simulink model "exampleThermalConductivity"  (Simulink 7.6)
settings: Solver=ode45  StartTime=0.0  StopTime=10.0  RelTol=1e-3
libraries: carnot x4
settings Model: Creator=drhf  LastModifiedBy=drhf

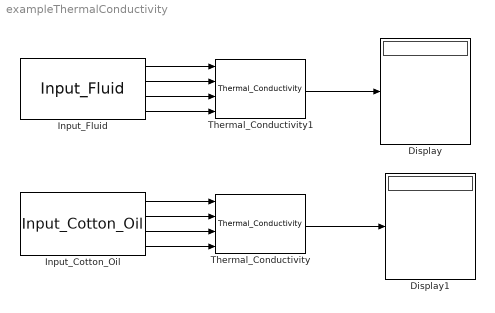
== system exampleThermalConductivity ==
  Display : Display
  Display1 : Display
  Input_Cotton_Oil : carnot/Basic/Material_Properties/Input_Cotton_Oil  SystemSampleTime=-1  T=[10:10:50]  p=1e5
  Input_Fluid : carnot/Basic/Material_Properties/Input_Fluid  SystemSampleTime=-1  fluid=water  T=[10:10:50]  p=1e5  x=0.005
  Thermal_Conductivity : carnot/Basic/Material_Properties/Thermal_Conductivity  SystemSampleTime=-1
  Thermal_Conductivity1 : carnot/Basic/Material_Properties/Thermal_Conductivity  SystemSampleTime=-1
  wires:
  Input_Fluid/1 -> Thermal_Conductivity1/1
  Input_Fluid/2 -> Thermal_Conductivity1/2
  Input_Fluid/3 -> Thermal_Conductivity1/3
  Input_Fluid/4 -> Thermal_Conductivity1/4
  Thermal_Conductivity1/1 -> Display/1
  Input_Cotton_Oil/1 -> Thermal_Conductivity/1
  Input_Cotton_Oil/2 -> Thermal_Conductivity/2
  Input_Cotton_Oil/3 -> Thermal_Conductivity/3
  Input_Cotton_Oil/4 -> Thermal_Conductivity/4
  Thermal_Conductivity/1 -> Display1/1
